simulink model "SwatchModel"  (R2014b)
settings: Solver=ode3  StartTime=0.0  StopTime=inf  FixedStep=0.1  RelTol=1e-3
libraries: simulink x1
settings Model: Creator=paolosassi  LastModifiedBy=paolosassi
settings OptimizationCC: InlineParams=on  InlineInvariantSignals=on  PassReuseOutputArgsAs=Individual arguments  OptimizeModelRefInitCode=on  LifeSpan=Inf
settings RTWCC: SystemTargetFile=ert.tlc  GenCodeOnly=on  TemplateMakefile=ert_default_tmf  Description=Embedded Coder  ProcessScript=ert_make_rtw_hook
settings CodeAppCC: IgnoreCustomStorageClasses=off
settings ERTTargetCC: IncludeMdlTerminateFcn=off  GeneratePreprocessorConditionals=Disable all  SupportAbsoluteTime=off  MultiInstanceERTCode=on  CodeInterfacePackaging=Reusable function  SupportNonFinite=off  SupportComplex=off  PurelyIntegerCode=on  MultiInstanceErrorCode=None  ERTCustomFileTemplate=example_file_process.tlc  IndentSize=4

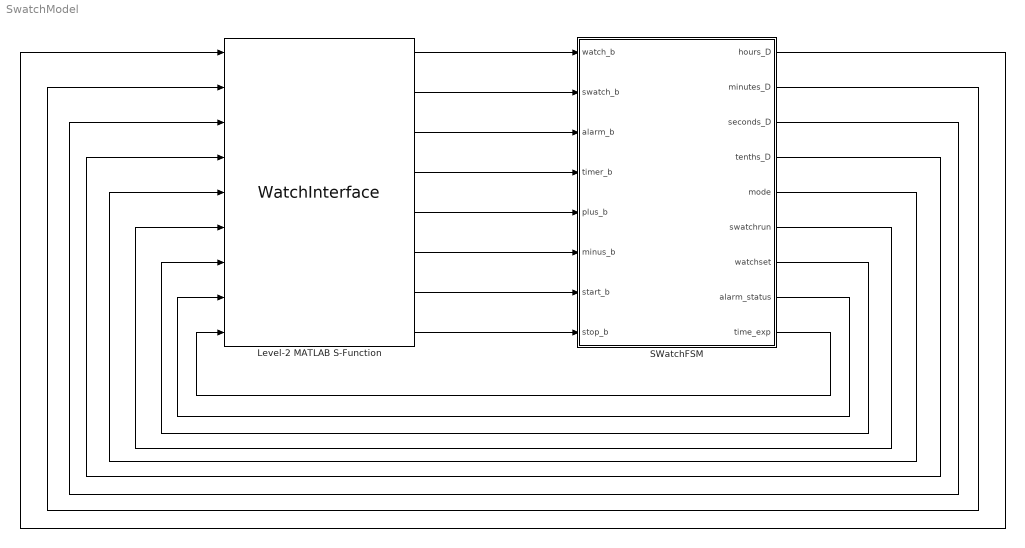
== system SwatchModel ==
  Level-2 MATLAB S-Function : M-S-Function  FunctionName=WatchInterface
  SWatchFSM : Subsystem
  wires:
  Level-2 MATLAB S-Function/1 -> SWatchFSM/1(watch_b)
  Level-2 MATLAB S-Function/2 -> SWatchFSM/2(swatch_b)
  Level-2 MATLAB S-Function/3 -> SWatchFSM/3(alarm_b)
  Level-2 MATLAB S-Function/4 -> SWatchFSM/4(timer_b)
  Level-2 MATLAB S-Function/5 -> SWatchFSM/5(plus_b)
  Level-2 MATLAB S-Function/6 -> SWatchFSM/6(minus_b)
  SWatchFSM/1(hours_D) -> Level-2 MATLAB S-Function/1
  SWatchFSM/2(minutes_D) -> Level-2 MATLAB S-Function/2
  SWatchFSM/3(seconds_D) -> Level-2 MATLAB S-Function/3
  SWatchFSM/4(tenths_D) -> Level-2 MATLAB S-Function/4
  SWatchFSM/5(mode) -> Level-2 MATLAB S-Function/5
  SWatchFSM/9(time_exp) -> Level-2 MATLAB S-Function/9
  SWatchFSM/8(alarm_status) -> Level-2 MATLAB S-Function/8
  SWatchFSM/7(watchset) -> Level-2 MATLAB S-Function/7
  SWatchFSM/6(swatchrun) -> Level-2 MATLAB S-Function/6
  Level-2 MATLAB S-Function/7 -> SWatchFSM/7(start_b)
  Level-2 MATLAB S-Function/8 -> SWatchFSM/8(stop_b)

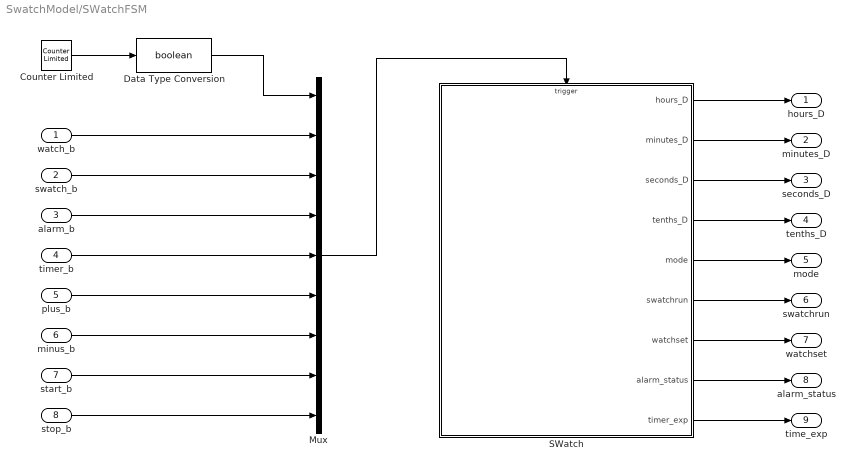
== system SwatchModel/SWatchFSM ==
  watch_b : Inport
  swatch_b : Inport  Port=2
  alarm_b : Inport  Port=3
  timer_b : Inport  Port=4
  plus_b : Inport  Port=5
  minus_b : Inport  Port=6
  start_b : Inport  Port=7
  stop_b : Inport  Port=8
  Counter Limited : simulink/Sources/Counter Limited  uplimit=1  tsamp=0.1
  Data Type Conversion : DataTypeConversion  OutDataTypeStr=boolean
  Mux : Mux  Inputs=9
  SWatch : Stateflow chart  TreatAsAtomicUnit=on
  hours_D : Outport
  minutes_D : Outport  Port=2
  seconds_D : Outport  Port=3
  tenths_D : Outport  Port=4
  mode : Outport  Port=5
  swatchrun : Outport  Port=6
  watchset : Outport  Port=7
  alarm_status : Outport  Port=8
  time_exp : Outport  Port=9
  wires:
  Mux/1 -> SWatch/Trigger
  alarm_b/1 -> Mux/4
  minus_b/1 -> Mux/7
  SWatch/6(swatchrun) -> swatchrun/1
  SWatch/4(tenths_D) -> tenths_D/1
  start_b/1 -> Mux/8
  SWatch/8(alarm_status) -> alarm_status/1
  SWatch/7(watchset) -> watchset/1
  SWatch/2(minutes_D) -> minutes_D/1
  SWatch/1(hours_D) -> hours_D/1
  plus_b/1 -> Mux/6
  watch_b/1 -> Mux/2
  SWatch/5(mode) -> mode/1
  SWatch/9(timer_exp) -> time_exp/1
  stop_b/1 -> Mux/9
  SWatch/3(seconds_D) -> seconds_D/1
  Data Type Conversion/1 -> Mux/1
  Counter Limited/1 -> Data Type Conversion/1
  timer_b/1 -> Mux/5
  swatch_b/1 -> Mux/3

== stateflow chart SwatchModel/SWatchFSM/SWatch ==
  settings: executeAtInitialization=1
  state Mode_mng [parallel]
    settings: executionOrder=1
    state watch_m
      en:mode = uint8(0)
      exit: watchset = uint8(0)
      state watch_showtime
      state watch_settime
        en: hours_D = hours_W;
        minutes_D = minutes_W;
        seconds_D = uint8(0);
        state watch_sethours
          en: hours_D = hours_W
        state watch_setminutes
          en: minutes_D = minutes_W
        watch_setminutes -> watch_setminutes [order 1] : plus_b{minutes_W = mod(minutes_W + 1,  60);}
        watch_sethours -> watch_sethours [order 2] : plus_b{hours_W = mod(hours_W + 1,  24);}
        (default) -> watch_sethours
        watch_sethours -> watch_setminutes [order 1] : watch_b
        watch_setminutes -> watch_setminutes [order 2] : minus_b{minutes_W = mod(minutes_W - 1, 60)}
        watch_sethours -> watch_sethours [order 3] : minus_b{hours_W = mod(hours_W - 1, 24)}
      watch_showtime -> watch_showtime [order 2] : tick_t{hours_D = hours_W;
          | minutes_D = minutes_W;
          | seconds_D = seconds_W;
          | tenths_D = tenths_W}
      (default) -> watch_showtime : {watchset = uint8(0);}
      watch_setminutes -> watch_showtime [order 3] : watch_b {seconds_W = uint8(0);
          | tenths_W = uint8(0);
          | watchset = uint8(0);}
      watch_showtime -> watch_settime [order 1] : watch_b{watchset = uint8(1);}
    state swatch_m
      en:mode = uint8(1);hours_D = hours_S; minutes_D = minutes_S;
      seconds_D = seconds_S; tenths_D = tenths_S;
      during: hours_D = hours_S; minutes_D = minutes_S;
      seconds_D = seconds_S; tenths_D = tenths_S;
      (history)
      state swatch_stop
      state swatch_running
      state swatch_pause
      (default) -> swatch_stop
      swatch_stop -> swatch_running : start_b{swatchrun = uint8(1)}
      swatch_pause -> swatch_running [order 1] : start_b{swatchrun = uint8(1)}
      swatch_pause -> swatch_stop [order 2] : stop_b{swatchrun = uint8(0);}
      swatch_running -> swatch_pause : stop_b{swatchrun = uint8(2)}
    state alarm_m
      en:mode = uint8(2);
      hours_D = hours_A;
      minutes_D = minutes_A;
      (history)
      state alarm_set
        en: hours_D = hours_A;
        minutes_D = minutes_A;
        state alarm_sethours
          en: hours_D = hours_A
        state alarm_setminutes
          en: minutes_D = minutes_A
        alarm_setminutes -> alarm_setminutes [order 2] : plus_b{minutes_A = mod(minutes_A + 1,  60);}
        alarm_sethours -> alarm_sethours [order 2] : plus_b{hours_A = mod(hours_A + 1,  24);}
        (default) -> alarm_sethours
        alarm_sethours -> alarm_setminutes [order 1] : alarm_b
        alarm_setminutes -> alarm_sethours [order 1] : alarm_b
        alarm_setminutes -> alarm_setminutes [order 3] : minus_b{minutes_A = mod(minutes_A - 1, 60);}
        alarm_sethours -> alarm_sethours [order 3] : minus_b{hours_A = mod(hours_A - 1, 24)}
      state alarm_running
      (default) -> alarm_set
      alarm_set -> alarm_running [order 1] : start_b[hours_A > hours_W || (hours_A == hours_W && minutes_A > minutes_W)]
          | {alarm_status = uint8(1);}
      alarm_set -> alarm_set [order 2] : stop_b{hours_A = uint8(0);
          | minutes_A = uint8(0)}
      alarm_running -> alarm_set [order 1] : tick_t[alarm_cycle == uint8(0)]
      alarm_running -> alarm_set [order 2] : stop_b{hours_A = uint8(0); minutes_A = uint8(0);
          | alarm_status = uint8(0);}
    state timer_m
      en:mode = uint8(3);
      hours_D = hours_T;
      minutes_D = minutes_T;
      seconds_D = seconds_T;
      (history)
      state timer_running
        during: hours_D = hours_T;
        minutes_D = minutes_T;
        seconds_D = seconds_T;
      state timer_set
        en: hours_D = hours_T;
        minutes_D = minutes_T;
        seconds_D = seconds_T;
        state timer_setminutes
          en: minutes_D = minutes_T
        state timer_sethours
          en: hours_D = hours_T
        state timer_setseconds
          en: seconds_D = seconds_T
        timer_setseconds -> timer_sethours [order 3] : timer_b
        timer_setminutes -> timer_setminutes [order 1] : plus_b{minutes_T = mod(minutes_T + 1,  60);}
        timer_sethours -> timer_sethours [order 2] : plus_b{hours_T = mod(hours_T + 1,  24);}
        timer_setseconds -> timer_setseconds [order 1] : plus_b{seconds_T = mod(seconds_T + 1,  60);}
        (default) -> timer_sethours
        timer_sethours -> timer_setminutes [order 1] : timer_b
        timer_setminutes -> timer_setseconds [order 3] : timer_b
        timer_setseconds -> timer_setseconds [order 2] : minus_b{seconds_T = mod(seconds_T - 1, 60);}
        timer_sethours -> timer_sethours [order 3] : minus_b{hours_T = mod(hours_T - 1, 24)}
        timer_setminutes -> timer_setminutes [order 2] : minus_b{minutes_T = mod(minutes_T - 1, 60);}
      timer_set -> timer_set [order 2] : stop_b{hours_T = uint8(0);
          | minutes_T = uint8(0);
          | seconds_T = uint8(0);
          | tenths_T = uint8(0);}
      (default) -> timer_set
      timer_running -> timer_set : stop_b{hours_T = uint8(0); minutes_T = uint8(0);
          |  seconds_T = uint8(0); tenths_T = uint8(0);
          | timer_exp = uint8(0);}
      timer_set -> timer_running [order 1] : start_b[hours_T > uint8(0) || (hours_T == uint8(0) && minutes_T > uint8(0)) || (hours_T == uint8(0) && minutes_T == uint8(0) && seconds_T > uint8(0))]
    (default) -> watch_m
    swatch_m -> watch_m [order 3] : watch_b
    Mode_mng -> swatch_m : swatch_b
    watch_m -> timer_m [order 1] : timer_b
    alarm_m -> watch_m [order 2] : watch_b
    watch_m -> alarm_m [order 2] : alarm_b
    timer_m -> watch_m [order 2] : watch_b
    swatch_m -> alarm_m [order 2] : alarm_b
    swatch_m -> timer_m [order 1] : timer_b
    alarm_m -> timer_m [order 1] : timer_b
    timer_m -> alarm_m [order 1] : alarm_b
  state Watch_mng [parallel]
    settings: executionOrder=2
    state W_count
    W_count -> (junction 38) : tick_t{tenths_W = mod(tenths_W + 1, 10)}
    (junction 38) -> (junction 39) [order 2]
    (junction 38) -> (junction 40) [order 1] : [tenths_W == 0]
        | {seconds_W = mod(seconds_W + 1, 60)}
    (default) -> W_count : {hours_W = uint8(0); minutes_W = uint8(0);
        | seconds_W = uint8(0); tenths_W = uint8(0)}
    (junction 39) -> W_count
    (junction 40) -> (junction 39) [order 2]
    (junction 41) -> (junction 39) [order 2]
    (junction 41) -> (junction 39) [order 1] : [minutes_W == 0]
        | {hours_W = mod(hours_W + 1,  24)}
    (junction 40) -> (junction 41) [order 1] : [seconds_W == 0]
        | {minutes_W = mod(minutes_W + 1,  60)}
  state Swatch_mng [parallel]
    settings: executionOrder=3
    state S_count
    state S_stop
    S_count -> (junction 71) [order 1] : tick_t{tenths_S = mod(tenths_S + 1, 10)}
    (junction 71) -> (junction 73) [order 2]
    (junction 71) -> (junction 74) [order 1] : [tenths_S == 0]
        | {seconds_S = mod(seconds_S + 1, 60)}
    (junction 73) -> S_count
    (junction 74) -> (junction 73) [order 2]
    (junction 75) -> (junction 73) [order 2]
    (junction 75) -> (junction 73) [order 1] : [minutes_S == 0]
        | {hours_S = mod(hours_S + 1,  24)}
    (junction 74) -> (junction 75) [order 1] : [seconds_S == 0]
        | {minutes_S = mod(minutes_S + 1,  60)}
    S_count -> S_stop [order 2] : stop_b[mode == uint8(1)]
    S_stop -> S_count [order 1] : start_b[mode == uint8(1)]
    (default) -> S_stop : {hours_S = uint8(0); minutes_S = uint8(0);
        | seconds_S = uint8(0); tenths_S = uint8(0)}
    S_stop -> S_stop [order 2] : stop_b[mode == uint8(1)]{hours_S = uint8(0);
        | minutes_S = uint8(0);
        | seconds_S = uint8(0);
        | tenths_S = uint8(0)}
  state Alarm_mng [parallel]
    settings: executionOrder=4
    state A_count
    state A_exp
    state A_stop
    A_exp -> A_exp [order 2] : tick_t[alarm_status == uint8(2)]
        | {alarm_status = uint8(1);
        | alarm_cycle = alarm_cycle - 1;}
    A_exp -> A_exp [order 3] : tick_t[alarm_status == uint8(1)]
        | {alarm_status = uint8(2);
        | alarm_cycle = alarm_cycle - 1;}
    A_count -> A_exp [order 1] : tick_t[minutes_W == minutes_A && hours_W == hours_A]
        | {alarm_status = uint8(2); }
    A_stop -> A_count : start_b[mode == uint8(2) && ...
        | (hours_A > hours_W || ...
        | (hours_A == hours_W && ...
        | minutes_A > minutes_W))]
    A_count -> A_stop [order 2] : stop_b[mode == uint8(2)]
    A_exp -> A_stop [order 1] : tick_t[alarm_status == uint8(0) || ...
        |  alarm_cycle == uint8(0)]
        | {alarm_cycle = uint8(200);}
    (default) -> A_stop : {hours_A = uint8(0);
        | minutes_A = uint8(0);
        | alarm_status = uint8(0);
        | alarm_cycle = uint8(200);}
  state Timer_mng [parallel]
    settings: executionOrder=5
    state T_count
    state T_stop
    T_count -> (junction 196) [order 2] : tick_t{tenths_T = tenths_T - uint8(1)}
    (junction 196) -> (junction 197) [order 2]
    (junction 196) -> (junction 290) [order 1] : [tenths_T == uint8(0)]
        | {tenths_T = uint8(9);}
    (junction 290) -> (junction 197) [order 1] : [seconds_T == uint8(1)]
        | {seconds_T = seconds_T - uint8(1);}
    (junction 290) -> (junction 198) [order 2] : {seconds_T = seconds_T - uint8(1);}
    (junction 197) -> T_count
    (junction 198) -> (junction 197) [order 3]
    (junction 287) -> (junction 197) [order 1] : [minutes_T == uint8(1)]
        | {minutes_T = minutes_T - uint8(1);}
    (junction 199) -> (junction 197) [order 1] : [minutes_T == uint8(0) && hours_T > uint8(0)]
        | {minutes_T = uint8(59);
        | hours_T = hours_T - uint8(1);}
    (junction 199) -> (junction 197) [order 2]
    T_stop -> T_count : start_b[mode == uint8(3) && (hours_T > uint8(0) || ...
        | (hours_T == uint8(0) && minutes_T > uint8(0)) || ...
        | (hours_T == uint8(0) && minutes_T == uint8(0) && ...
        | seconds_T > uint8(0)))]
    T_count -> T_stop [order 1] : stop_b[mode == uint8(3)]
    (junction 198) -> T_stop [order 1] : [seconds_T == uint8(0) && ...
        | minutes_T == uint8(0) && ...
        | hours_T == uint8(0)]
        | {timer_exp = uint8(1);}
    (junction 198) -> (junction 287) [order 2] : [seconds_T == uint8(0)]
        | {seconds_T = uint8(59);}
    (default) -> T_stop : {hours_T = uint8(0); minutes_T = uint8(0);
        | seconds_T = uint8(0); tenths_T = uint8(0);
        |  timer_exp = uint8(0);}
    (junction 287) -> (junction 199) [order 2] : {minutes_T = minutes_T - uint8(1);}
  data: hours_D output uint8; minutes_D output uint8; seconds_D output uint8; tenths_D output uint8; mode output uint8; hours_W local uint8; minutes_W local uint8; seconds_W local uint8; tenths_W local uint8; hours_S local uint8; minutes_S local uint8; seconds_S local uint8; tenths_S local uint8; swatchrun output uint8; watchset output uint8; minutes_A local uint8; hours_A local uint8; tenths_T local uint8; seconds_T local uint8; minutes_T local uint8; hours_T local uint8; alarm_status output uint8; timer_exp output uint8; alarm_cycle local uint8
  events: tick_t input EITHER_EDGE_EVENT; watch_b input RISING_EDGE_EVENT; swatch_b input RISING_EDGE_EVENT; alarm_b input RISING_EDGE_EVENT; timer_b input RISING_EDGE_EVENT; plus_b input RISING_EDGE_EVENT; minus_b input RISING_EDGE_EVENT; start_b input RISING_EDGE_EVENT; stop_b input RISING_EDGE_EVENT
